simulink model "Kalman"  (R2015a)
settings: Solver=ode2  StartTime=0.0  StopTime=10.0  FixedStep=0.01  RelTol=1e-3
settings Model: Creator=pela  LastModifiedBy=Mattia
settings HardwareCC: ProdLargestAtomicInteger=Long  ProdLargestAtomicFloat=Double  ProdIntDivRoundTo=Zero  ProdEndianess=LittleEndian  ProdHWDeviceType=ARM Compatible->ARM Cortex
settings RTWCC: GenCodeOnly=on  GenerateReport=on  Toolchain=Microsoft Visual C++ 2013 v12.0 | nmake (64-bit Windows)  BuildConfiguration=Faster Runs  LaunchReport=on  TargetLang=C++
settings GRTTargetCC: MatFileLogging=off  MultiInstanceERTCode=on  CodeInterfacePackaging=C++ class  SupportNonFinite=off

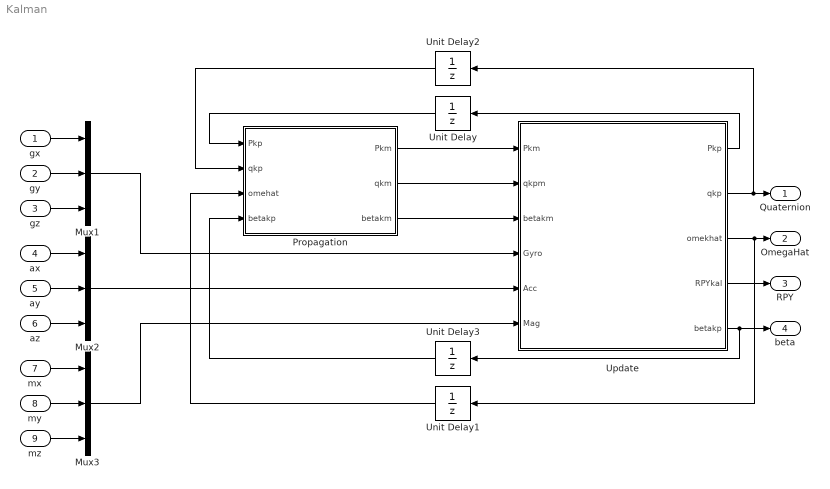
== system Kalman ==
  gx : Inport
  gy : Inport  Port=2
  gz : Inport  Port=3
  ax : Inport  Port=4
  ay : Inport  Port=5
  az : Inport  Port=6
  mx : Inport  Port=7
  my : Inport  Port=8
  mz : Inport  Port=9
  Mux1 : Mux  Inputs=3
  Mux2 : Mux  Inputs=3
  Mux3 : Mux  Inputs=3
  "Propagation " : MATLAB Function  TreatAsAtomicUnit=on
  Unit Delay : UnitDelay  InitialCondition=(1e-6)*[1 0 0 0 0 0; 0 1 0 0 0 0; 0 0 1 0 0 0; 0 0 0 1 0 0; 0 0 0 0 1 0; 0 0 0 0 0 1]  SampleTime=-1
  Unit Delay1 : UnitDelay  InitialCondition=0.00001*[1 1 1]'  SampleTime=-1
  Unit Delay2 : UnitDelay  InitialCondition=[0 0 0 1]'  SampleTime=-1
  Unit Delay3 : UnitDelay  InitialCondition=0.00001*[1 1 1]'  SampleTime=-1
  Update : MATLAB Function  TreatAsAtomicUnit=on
  Quaternion : Outport
  OmegaHat : Outport  Port=2
  RPY : Outport  Port=3
  "beta " : Outport  Port=4
  wires:
  Update/1(Pkp) -> Unit Delay/1
  Update/3(omekhat) -> Unit Delay1/1, OmegaHat/1
  Unit Delay1/1 -> "Propagation "/3(omehat)
  Unit Delay/1 -> "Propagation "/1(Pkp)
  "Propagation "/1(Pkm) -> Update/1(Pkm)
  gx/1 -> Mux1/1
  gy/1 -> Mux1/2
  ax/1 -> Mux2/1
  mx/1 -> Mux3/1
  az/1 -> Mux2/3
  Update/2(qkp) -> Unit Delay2/1, Quaternion/1
  Update/5(betakp) -> Unit Delay3/1, "beta "/1
  gz/1 -> Mux1/3
  ay/1 -> Mux2/2
  Unit Delay2/1 -> "Propagation "/2(qkp)
  "Propagation "/2(qkm) -> Update/2(qkpm)
  mz/1 -> Mux3/3
  my/1 -> Mux3/2
  Mux1/1 -> Update/4(Gyro)
  Mux2/1 -> Update/5(Acc)
  Mux3/1 -> Update/6(Mag)
  Unit Delay3/1 -> "Propagation "/4(betakp)
  Update/4(RPYkal) -> RPY/1
  "Propagation "/3(betakm) -> Update/3(betakm)

== matlab function Kalman/Update ==
  data Pkm settings: description=A-priori state estimate.
  data qkpm settings: description=A-priori covariance estimate.
  data betakm settings: description=Measurements from the sensors.
  data Pkp settings: description=Corrected state estimate.
  data omekhat settings: description=Corrected covariance estimate.
  data: Pkm input; qkpm input; betakm input; Gyro input; Pkp output; qkp output; omekhat output; RPYkal output; Acc input; Mag input; betakp output
%% EKF - Update           %
% Author: Mattia Giurato  %
% Last review: 2016/03/15 %
%%%%%%%%%%%%%%%%%%%%%%%%%%%
function [Pkp,qkp,omekhat,RPYkal,betakp] = Update(Pkm,qkpm,betakm,Gyro,Acc,Mag)
gx = Gyro(1);
gy = Gyro(2);
gz = Gyro(3);
ax = Acc(1);
ay = Acc(2);
az = Acc(3);
mx = Mag(1);
my = Mag(2);
mz = Mag(3);
Gyroscope = [gx gy gz]';
Accelerometer = [ax ay az]';
Magnetometer = [mx my mz]';

% Usefull values
sigma_acc = diag([0.77418 0.66936 0.71485]);
sigma_mag = 300*diag([0.053667 0.034382 0.071054]);
I3 = [1 0 0; 0 1 0; 0 0 1];
I6 = [1 0 0 0 0 0; 0 1 0 0 0 0; 0 0 1 0 0 0; 0 0 0 1 0 0; 0 0 0 0 1 0; 0 0 0 0 0 1];
O3 = [0 0 0; 0 0 0; 0 0 0];

% Normalise accelerometer measurement
b_acc = Accelerometer / sqrt(ax^2 + ay^2 + az^2); % normalise magnitude

% Normalise magnetometer measurement
b_mag = Magnetometer / sqrt(mx^2 + my^2 + mz^2); % normalise magnitude

%% Propagated value from previous step
deltaXkm = zeros(6,1);

%% Accelerometer and Magnetometer correction
% Compute attitude matrix
ro = [qkpm(1) ;
      qkpm(2) ;
      qkpm(3)];
q_4 = qkpm(4);
rox = [   0   -ro(3)  ro(2) ;
         ro(3)  0    -ro(1) ;
        -ro(2) ro(1)   0   ];
norm_ro_sq = ro(1)^2 + ro(2)^2 + ro(3)^2;
Aqkm = (q_4^2 - norm_ro_sq)*I3 + 2*(ro*ro') - 2*q_4*rox;
% Reference direction of Earth's gravitational field
r_acc = [0 ;
         0 ;
         1];
Aqmr = Aqkm*r_acc;
b = b_acc;
R = sigma_acc^2*I3;

% Sensitivity Matrix
Aqmrx = [   0     -Aqmr(3)  Aqmr(2) ;
          Aqmr(3)    0     -Aqmr(1) ;
         -Aqmr(2)  Aqmr(1)    0    ];
Hk = [Aqmrx O3];

% Gain
Kk = (Pkm*Hk')/(Hk*Pkm*Hk' + R);

% Update Covariance
Pkp = (I6 - Kk*Hk)*Pkm*(I6 - Kk*Hk)' + Kk*R*Kk';

% Update state
epk = b - Aqmr; %residual
yk = epk - Hk*deltaXkm;
deltaXkp = (deltaXkm + Kk*yk);

Pkm = Pkp;
deltaXkm = deltaXkp;

% Reference direction of Earth's magnetic feild
h = Aqkm*Magnetometer;
norm_h = sqrt(h(1)^2 + h(2)^2);
r_mag = [norm_h ;
           0    ;
          h(3) ];
Aqmr = Aqkm*r_mag;
b = b_mag;
R = sigma_mag^2*I3;

% Sensitivity Matrix
Aqmrx = [      0   -Aqmr(3)  Aqmr(2) ;
           Aqmr(3)    0     -Aqmr(1) ;
          -Aqmr(2)  Aqmr(1)    0    ];
Hk = [Aqmrx O3];

% Gain
Kk = (Pkm*Hk')/(Hk*Pkm*Hk' + R);

% Update Covariance
Pkp = (I6 - Kk*Hk)*Pkm*(I6 - Kk*Hk)' + Kk*R*Kk';

% Update state
epk = b - Aqmr; %residual
yk = epk - Hk*deltaXkm;
deltaXkp = (deltaXkm + Kk*yk);

% Update quaternion
dalphak = deltaXkp(1:3,1);
norm_dalphak_sq = dalphak(1)^2 + dalphak(2)^2 + dalphak(3)^2;
dq = (1/sqrt(4+norm_dalphak_sq))*[dalphak' 2]';
qkp = [dq(4)*ro + q_4*dq(1:3,1)-cross(dq(1:3,1),ro) ;
               dq(4)*q_4 - dot(dq(1:3,1),ro)       ];

% Update biases
deltaBeta = deltaXkp(4:6,1);
betakp = betakm + deltaBeta;
  
%% Depolarize gyroscope measurement
omekhat = Gyroscope - betakp;

%% Convert Quaternion into RPY
a1 = 2.*(qkp(1).*qkp(2) + qkp(4).*qkp(3));
a2 = qkp(4).^2 + qkp(1).^2 - qkp(2).^2 - qkp(3).^2;
b = -2.*(qkp(1).*qkp(3) - qkp(4).*qkp(2));
c1 = 2.*(qkp(2).*qkp(3) + qkp(4).*qkp(1));
c2 = qkp(4).^2 - qkp(1).^2 - qkp(2).^2 + qkp(3).^2;

Yy = atan2(a1, a2);
Pp = asin(b);
Rr = atan2(c1, c2);

RPYkal = [Rr -Pp -Yy]';

== matlab function Kalman/Propagation  ==
  data Pkp settings: description=Control signal at the previous step.
  data qkp settings: description=Covariance estimate at the previous step.
  data Pkm settings: description=A-priori covariance estimate.
  data qkm settings: description=A-priori state estimate.
  data: Pkp input; qkp input; Pkm output; qkm output; omehat input; betakp input; betakm output
%% EKF - Propagation      %
% Author: Mattia Giurato  %
% Last review: 2016/03/15 %
%%%%%%%%%%%%%%%%%%%%%%%%%%%
function [Pkm,qkm,betakm] = Propagation(Pkp,qkp,omehat,betakp)
%% Usefull values
sigma_u = diag([0.13807 0.11053 0.063833/10])/100;
sigma_v = diag([0.00001 0.00001 0.05]);
dt = 0.01;
I3 = [1 0 0; 0 1 0; 0 0 1];
O3 = [0 0 0; 0 0 0; 0 0 0];

%% Quaternion propagation
omex = [     0      -omehat(3)  omehat(2) ;
         omehat(3)      0      -omehat(1) ;
        -omehat(2)  omehat(1)      0     ];
Omega = [ -omex   omehat ;
         -omehat'     0 ];
qt = (eye(4) + .5*Omega*dt)*qkp;
qkm = qt / sqrt(qt(1)^2+qt(2)^2+qt(3)^2+qt(4)^2);

%% Bias propagation
betakm = betakp; 

%% Covariance equation propagation
Phi1 = I3;
Phi2 = -I3*dt;
Phi = [Phi1 Phi2 ;
        O3   I3 ];
gamma = [-I3 O3 ;
          O3 I3];
Q = [(sigma_v^2*dt + 1/3*sigma_u^2*dt^3)*I3 (.5*sigma_u^2*dt^2)*I3 ;
             (.5*sigma_u^2*dt^2)*I3            (sigma_u^2*dt)*I3  ];
Pkm = Phi*Pkp*Phi' + gamma*Q*gamma';
